simulink model "OML58_Cores"  (R2021b)
settings: Solver=ode4  StartTime=0.0  StopTime=inf  FixedStep=Ts  RelTol=1e-3  EnableMultiTasking=on
PostLoadFcn:
  | Ts = 50e-6;
InitFcn:
  | Ts = 50e-6;
undefined symbols (not defined in the file): I, Left, Right, type, V
libraries: spsSeriesRLCBranchLib x24, spsThreePhaseSeriesRLCLoadLib x12, spsThreePhaseSeriesRLCBranchLib x12, spsThreePhaseBreakerLib x12, artemis x10, spsGroundLib x8, rtlab x6, LafaeLib x6, spsThreePhaseTransformerTwoWindingsLib x5, spsThreePhaseVIMeasurementLib x5, spsPower3phInstantaneousLib x3, spsThreePhaseSourceLib x1
(part 2 of 3)

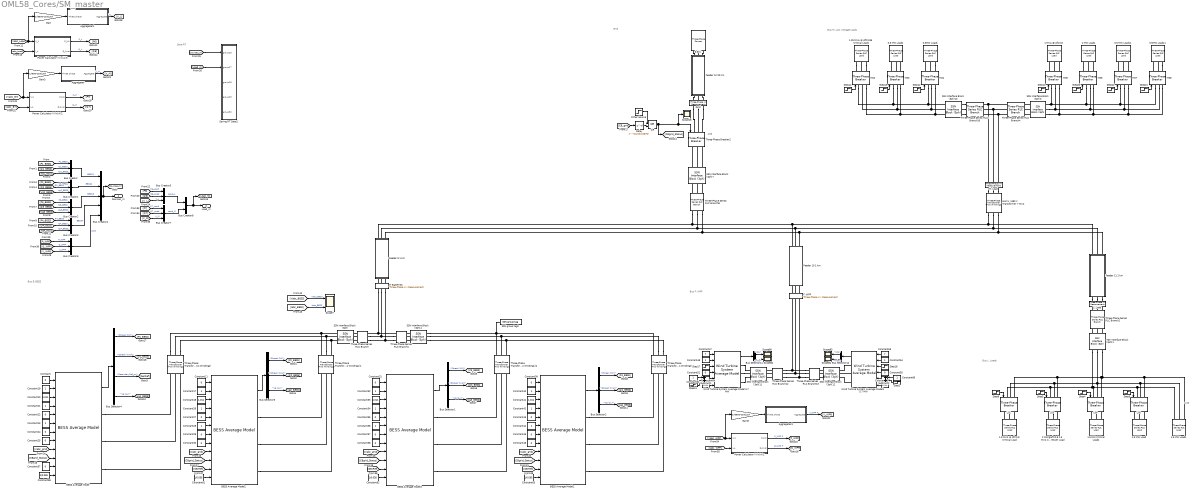
== system OML58_Cores/SM_master ==
  note: Bus E: BESS
  note: L06
  note: Bus L: Loads
  note: Save RT
  note: Grid
  note: A06
  note: Bus M: Low Voltage Loads
  note: Bus F: WPP
  0.5 MW Loads : spsThreePhaseSeriesRLCLoadLib/Three-Phase Series RLC Load  LConnTagsString=A|B|C  Configuration=Y (grounded)  NominalVoltage=690  Vabc=[1e3 1e3 1e3]  Vabcp=[1e3 1e3 1e3]  NominalFrequency=50  UnbalancedPower=off  ActivePower=0.5e06  InductivePower=0  CapacitivePower=0  Pabc=[10e3 9e3 11e3]  QLabc=[100 90 110]  QCabc=[100 90 110]  Pabcp=[10e3 9e3 11e3]  QLabcp=[100 90 110]  QCabcp=[100 90 110]  Measurements=None  LoadType=constant Z
  0.5 MW Loads1 : spsThreePhaseSeriesRLCLoadLib/Three-Phase Series RLC Load  LConnTagsString=A|B|C  Configuration=Y (grounded)  NominalVoltage=690  Vabc=[1e3 1e3 1e3]  Vabcp=[1e3 1e3 1e3]  NominalFrequency=50  UnbalancedPower=off  ActivePower=0.5e06  InductivePower=0  CapacitivePower=0  Pabc=[10e3 9e3 11e3]  QLabc=[100 90 110]  QCabc=[100 90 110]  Pabcp=[10e3 9e3 11e3]  QLabcp=[100 90 110]  QCabcp=[100 90 110]  Measurements=None  LoadType=constant Z
  0.5MW Loads : spsThreePhaseSeriesRLCLoadLib/Three-Phase Series RLC Load  LConnTagsString=A|B|C  Configuration=Y (grounded)  NominalVoltage=690  Vabc=[1e3 1e3 1e3]  Vabcp=[1e3 1e3 1e3]  NominalFrequency=50  UnbalancedPower=off  ActivePower=0.5e06  InductivePower=0  CapacitivePower=0  Pabc=[10e3 9e3 11e3]  QLabc=[100 90 110]  QCabc=[100 90 110]  Pabcp=[10e3 9e3 11e3]  QLabcp=[100 90 110]  QCabcp=[100 90 110]  Measurements=None  LoadType=constant Z
  0.5MW Loads1 : spsThreePhaseSeriesRLCLoadLib/Three-Phase Series RLC Load  LConnTagsString=A|B|C  Configuration=Y (grounded)  NominalVoltage=690  Vabc=[1e3 1e3 1e3]  Vabcp=[1e3 1e3 1e3]  NominalFrequency=50  UnbalancedPower=off  ActivePower=0.5e06  InductivePower=0  CapacitivePower=0  Pabc=[10e3 9e3 11e3]  QLabc=[100 90 110]  QCabc=[100 90 110]  Pabcp=[10e3 9e3 11e3]  QLabcp=[100 90 110]  QCabcp=[100 90 110]  Measurements=None  LoadType=constant Z
  1 MVA @ pf=0.8 : spsThreePhaseSeriesRLCLoadLib/Three-Phase Series RLC Load  LConnTagsString=A|B|C  Configuration=Y (grounded)  NominalVoltage=690  Vabc=[1e3 1e3 1e3]  Vabcp=[1e3 1e3 1e3]  NominalFrequency=50  UnbalancedPower=off  ActivePower=0.8e06  InductivePower=0.6e06  CapacitivePower=0  Pabc=[10e3 9e3 11e3]  QLabc=[100 90 110]  QCabc=[100 90 110]  Pabcp=[10e3 9e3 11e3]  QLabcp=[100 90 110]  QCabcp=[100 90 110]  Measurements=None  LoadType=constant Z
  1 MW Loads : spsThreePhaseSeriesRLCLoadLib/Three-Phase Series RLC Load  LConnTagsString=A|B|C  Configuration=Y (grounded)  NominalVoltage=690  Vabc=[1e3 1e3 1e3]  Vabcp=[1e3 1e3 1e3]  NominalFrequency=50  UnbalancedPower=off  ActivePower=0.5e06  InductivePower=0  CapacitivePower=0  Pabc=[10e3 9e3 11e3]  QLabc=[100 90 110]  QCabc=[100 90 110]  Pabcp=[10e3 9e3 11e3]  QLabcp=[100 90 110]  QCabcp=[100 90 110]  Measurements=None  LoadType=constant Z
  1.25 MVA @ pf=0.85 Critical Loads : spsThreePhaseSeriesRLCLoadLib/Three-Phase Series RLC Load  LConnTagsString=A|B|C  Configuration=Y (grounded)  NominalVoltage=690  Vabc=[1e3 1e3 1e3]  Vabcp=[1e3 1e3 1e3]  NominalFrequency=50  UnbalancedPower=off  ActivePower=1.0625e06  InductivePower=658478  CapacitivePower=0  Pabc=[10e3 9e3 11e3]  QLabc=[100 90 110]  QCabc=[100 90 110]  Pabcp=[10e3 9e3 11e3]  QLabcp=[100 90 110]  QCabcp=[100 90 110]  Measurements=None  LoadType=constant Z
  1.5 MW Critical Loads : spsThreePhaseSeriesRLCLoadLib/Three-Phase Series RLC Load  LConnTagsString=A|B|C  Configuration=Y (grounded)  NominalVoltage=6600  Vabc=[1e3 1e3 1e3]  Vabcp=[1e3 1e3 1e3]  NominalFrequency=50  UnbalancedPower=off  ActivePower=1.5e06  InductivePower=0  CapacitivePower=0  Pabc=[10e3 9e3 11e3]  QLabc=[100 90 110]  QCabc=[100 90 110]  Pabcp=[10e3 9e3 11e3]  QLabcp=[100 90 110]  QCabcp=[100 90 110]  Measurements=None  LoadType=constant Z
  1.5 MW Load : spsThreePhaseSeriesRLCLoadLib/Three-Phase Series RLC Load  LConnTagsString=A|B|C  Configuration=Y (grounded)  NominalVoltage=6600  Vabc=[1e3 1e3 1e3]  Vabcp=[1e3 1e3 1e3]  NominalFrequency=50  UnbalancedPower=off  ActivePower=1.5e06  InductivePower=0  CapacitivePower=0  Pabc=[10e3 9e3 11e3]  QLabc=[100 90 110]  QCabc=[100 90 110]  Pabcp=[10e3 9e3 11e3]  QLabcp=[100 90 110]  QCabcp=[100 90 110]  Measurements=None  LoadType=constant Z
  1.5 MW Loads : spsThreePhaseSeriesRLCLoadLib/Three-Phase Series RLC Load  LConnTagsString=A|B|C  Configuration=Y (grounded)  NominalVoltage=6600  Vabc=[1e3 1e3 1e3]  Vabcp=[1e3 1e3 1e3]  NominalFrequency=50  UnbalancedPower=off  ActivePower=1.5e06  InductivePower=0  CapacitivePower=0  Pabc=[10e3 9e3 11e3]  QLabc=[100 90 110]  QCabc=[100 90 110]  Pabcp=[10e3 9e3 11e3]  QLabcp=[100 90 110]  QCabcp=[100 90 110]  Measurements=None  LoadType=constant Z
  1.9 MVA @ pf=0.9 Critical Load : spsThreePhaseSeriesRLCLoadLib/Three-Phase Series RLC Load  LConnTagsString=A|B|C  Configuration=Y (grounded)  NominalVoltage=6600  Vabc=[1e3 1e3 1e3]  Vabcp=[1e3 1e3 1e3]  NominalFrequency=50  UnbalancedPower=off  ActivePower=1.71e06  InductivePower=828191  CapacitivePower=0  Pabc=[10e3 9e3 11e3]  QLabc=[100 90 110]  QCabc=[100 90 110]  Pabcp=[10e3 9e3 11e3]  QLabcp=[100 90 110]  QCabcp=[100 90 110]  Measurements=None  LoadType=constant Z
  2 MW@pf=0.8 2.5 MVA Compresser Load : spsThreePhaseSeriesRLCLoadLib/Three-Phase Series RLC Load  LConnTagsString=A|B|C  Configuration=Y (grounded)  NominalVoltage=6600  Vabc=[1e3 1e3 1e3]  Vabcp=[1e3 1e3 1e3]  NominalFrequency=50  UnbalancedPower=off  ActivePower=2e06  InductivePower=1.5e06  CapacitivePower=0  Pabc=[10e3 9e3 11e3]  QLabc=[100 90 110]  QCabc=[100 90 110]  Pabcp=[10e3 9e3 11e3]  QLabcp=[100 90 110]  QCabcp=[100 90 110]  Measurements=None  LoadType=constant Z
  "6.6 kV / 690 V Transformer 7 MVA   " : spsThreePhaseTransformerTwoWindingsLib/Three-Phase Transformer (Two Windings)  Winding1Connection=Yg  Winding2Connection=Yg  CoreType=Three single-phase transformers  SetSaturation=off  Hysteresis=off  DataFile='hysteresis'  SetInitialFlux=off  Measurements=None  UNITS=pu  NominalPower=[ 7e6 , 50 ]  Winding1=[ 6.6e3 , 0.03/25 , 0.03 ]  Winding2=[ 690 , 0.03/25 , 0.03 ]  Rm=500  Lm=500  L0=0.5  Saturation=[ 0,0 ; 0.0024,1.2 ; 1.0,1.52 ]  InitialFluxes=[ 0.8 , -0.8 , 0.7 ]  BreakLoop=off  DiscreteSolver=Trapezoidal iterative  DataType=off  TransfoNumber=1
  6.6kV : spsThreePhaseSourceLib/Three-Phase Source  InternalConnection=Yg  VoltagePhases=off  Voltage=6.6e3  PhaseAngle=0  Voltage_phases=[25e3 25e3 25e3]/sqrt(3)  PhaseAngles_phases=[0 -120 +120]  Frequency=50  NonIdealSource=on  SpecifyImpedance=on  Resistance=0.8929  Inductance=16.58e-3  ShortCircuitLevel=50e6*10  BaseVoltage=6.6e3  XRratio=7  BusType=swing  Pref=0  Qref=0  Prefabc=[10e3, 10e3, 10e3]  Qrefabc=[0, 0, 0]  Qmin=-inf  Qmax=inf
  Aggregater : Subsystem
      mask Display: image('$imagefile'); % Use "Edit Image" on toolstrip to change.
  Aggregater1 : Subsystem
      mask Display: image('$imagefile'); % Use "Edit Image" on toolstrip to change.
  Aggregater3 : Subsystem
      mask Display: image('$imagefile'); % Use "Edit Image" on toolstrip to change.
  BESS Average Model : LafaeLib/BESS/BESS Average Model  Vac=690  Vdc=1500  Snom=2.2e6  fnom=50  Capacity=1533  f_switch=6300  fres=720  Ripple=0.05  Kq=0.5  Kv=0.5/0.035  H=0.1  EnbSec=Yes  Ts=Ts
      settings: SourceProductName=LAFAE Library
  BESS Average Model1 : LafaeLib/BESS/BESS Average Model  Vac=690  Vdc=1500  Snom=2.2e6  fnom=50  Capacity=1533  f_switch=6300  fres=720  Ripple=0.05  Kq=0.5  Kv=0.5/0.035  H=0.1  EnbSec=No  Ts=Ts
      settings: SourceProductName=LAFAE Library
  BESS Average Model2 : LafaeLib/BESS/BESS Average Model  Vac=690  Vdc=1500  Snom=2.2e6  fnom=50  Capacity=1533  f_switch=6300  fres=720  Ripple=0.05  Kq=0.5  Kv=0.5/0.035  H=0.1  EnbSec=No  Ts=Ts
      settings: SourceProductName=LAFAE Library
  BESS Average Model3 : LafaeLib/BESS/BESS Average Model  Vac=690  Vdc=1500  Snom=2.2e6  fnom=50  Capacity=1533  f_switch=6300  fres=720  Ripple=0.05  Kq=0.5  Kv=0.5/0.035  H=0.1  EnbSec=No  Ts=Ts
      settings: SourceProductName=LAFAE Library
  Bus Creator{,1..3,5..7} (7 alike) : BusCreator  Inputs=3
  Bus Creator4 : BusCreator  Inputs=5
  Bus Creator8 : BusCreator  Inputs=2
  Bus Selector1 : BusSelector  OutputSignals=Pbreak (kW),Qbreak (kvar),Vg (pu)
  Bus Selector11 : BusSelector  OutputSignals=meas_control.Idq,meas_control.Vdq
  Bus Selector12 : BusSelector  OutputSignals=meas_control.Idq,meas_control.Vdq
  Bus Selector2 : BusSelector  OutputSignals=Pbreak (kW),Qbreak (kvar),Vg (pu)
  Bus Selector4 : BusSelector  OutputSignals=Pbreak (kW),Qbreak (kvar),SecondaryRef_pu,Vg (pu)
  Bus Selector5 : BusSelector  OutputSignals=Pbreak (kW),Qbreak (kvar),Vg (pu)
  Constant{,11,22,24..25,27,29..31,35,37..39,43,45..46,51,55,57} (19 alike) : Constant  Value=0
  Constant{17,19,21,23,26,28,32,34,36,40,42,44,48,52,54,66} (16 alike) : Constant
  Constant{18,20,33,41,64..65} (6 alike) : Constant  Value=1.011
  Constant47 : Constant  Value=7
  Constant53 : Constant  Value=7
  Constant{58,61..63} (4 alike) : Constant  Value=1/0.035
  Delay : Delay  DelayLength=round(0.05/Ts)  SampleTime=Ts
  E: Batteries : spsThreePhaseVIMeasurementLib/Three-Phase V-I Measurement  VoltageMeasurement=phase-to-ground  SetLabelV=on  LabelV=Vabc_BESS  Vpu=off  VpuLL=off  CurrentMeasurement=yes  SetLabelI=on  LabelI=Iabc_BESS  Ipu=off  Pbase=100e6  Vbase=500e3  OutputType=Magnitude  PhasorSimulation=off  PSBequivalent=0
  F: WPP : spsThreePhaseVIMeasurementLib/Three-Phase V-I Measurement  VoltageMeasurement=phase-to-ground  SetLabelV=on  LabelV=Vabc_WPP  Vpu=off  VpuLL=off  CurrentMeasurement=yes  SetLabelI=on  LabelI=Iabc_WPP  Ipu=off  Pbase=100e6  Vbase=500e3  OutputType=Magnitude  PhasorSimulation=off  PSBequivalent=0
  Feeder 10 1 km : Subsystem  mask{l=1}
      mask prompts: l "Comprimento da linha (km)"
      mask DialogControl DescTextVar Prompt: Modelo pi para sequência positiva.
      mask Display: image('$imagefile'); % Use "Edit Image" on toolstrip to change.
  Feeder 11 1 km : Subsystem  mask{l=1}
      mask prompts: l "Comprimento da linha (km)"
      mask DialogControl DescTextVar Prompt: Modelo pi para sequência positiva.
      mask Display: image('$imagefile'); % Use "Edit Image" on toolstrip to change.
  Feeder 12 20 km : Subsystem  mask{l=20}
      mask prompts: l "Comprimento da linha (km)"
      mask DialogControl DescTextVar Prompt: Modelo pi para sequência positiva.
      mask Display: image('$imagefile'); % Use "Edit Image" on toolstrip to change.
  Feeder 9 1 km : Subsystem  mask{l=1}
      mask prompts: l "Comprimento da linha (km)"
      mask DialogControl DescTextVar Prompt: Modelo pi para sequência positiva.
      mask Display: image('$imagefile'); % Use "Edit Image" on toolstrip to change.
  Gain : Gain  Gain=1/(6600*sqrt(2/3))
  Gain3 : Gain  Gain=1/(690*sqrt(2/3))
  Gain8 : Gain  Gain=1/(6600*sqrt(2/3))
  Grid : spsThreePhaseVIMeasurementLib/Three-Phase V-I Measurement  VoltageMeasurement=phase-to-ground  SetLabelV=on  LabelV=Vabc_grid  Vpu=off  VpuLL=off  CurrentMeasurement=yes  SetLabelI=on  LabelI=Iabc_grid  Ipu=off  Pbase=100e6  Vbase=500e3  OutputType=Magnitude  PhasorSimulation=off  PSBequivalent=0
  L02 : spsThreePhaseBreakerLib/Three-Phase Breaker  InitialState=open  SwitchA=on  SwitchB=on  SwitchC=on  SwitchTimes="[1/60  5/60]"  External=on  BreakerResistance=0.01  SnubberResistance=1e8  SnubberCapacitance=inf  Measurements=None
  L03 : spsThreePhaseBreakerLib/Three-Phase Breaker  InitialState=open  SwitchA=on  SwitchB=on  SwitchC=on  SwitchTimes="[1/60  5/60]"  External=on  BreakerResistance=0.01  SnubberResistance=1e8  SnubberCapacitance=inf  Measurements=None
  L04 : spsThreePhaseBreakerLib/Three-Phase Breaker  InitialState=open  SwitchA=on  SwitchB=on  SwitchC=on  SwitchTimes="[1/60  5/60]"  External=on  BreakerResistance=0.01  SnubberResistance=1e8  SnubberCapacitance=inf  Measurements=None
  L05 : spsThreePhaseBreakerLib/Three-Phase Breaker  InitialState=open  SwitchA=on  SwitchB=on  SwitchC=on  SwitchTimes="[1/60  5/60]"  External=on  BreakerResistance=0.01  SnubberResistance=1e8  SnubberCapacitance=inf  Measurements=None
  L: Load : spsThreePhaseVIMeasurementLib/Three-Phase V-I Measurement  VoltageMeasurement=phase-to-ground  SetLabelV=on  LabelV=Vabc_Load  Vpu=off  VpuLL=off  CurrentMeasurement=yes  SetLabelI=on  LabelI=Iabc_Load  Ipu=off  Pbase=100e6  Vbase=500e3  OutputType=Magnitude  PhasorSimulation=off  PSBequivalent=0
  M02 : spsThreePhaseBreakerLib/Three-Phase Breaker  InitialState=open  SwitchA=on  SwitchB=on  SwitchC=on  SwitchTimes="[1/60  5/60]"  External=on  BreakerResistance=0.01  SnubberResistance=1e7  SnubberCapacitance=inf  Measurements=None
  M03 : spsThreePhaseBreakerLib/Three-Phase Breaker  InitialState=open  SwitchA=on  SwitchB=on  SwitchC=on  SwitchTimes="[1/60  5/60]"  External=on  BreakerResistance=0.01  SnubberResistance=1e7  SnubberCapacitance=inf  Measurements=None
  M04 : spsThreePhaseBreakerLib/Three-Phase Breaker  InitialState=open  SwitchA=on  SwitchB=on  SwitchC=on  SwitchTimes="[1/60  5/60]"  External=on  BreakerResistance=0.01  SnubberResistance=1e7  SnubberCapacitance=inf  Measurements=None
  M05 : spsThreePhaseBreakerLib/Three-Phase Breaker  InitialState=open  SwitchA=on  SwitchB=on  SwitchC=on  SwitchTimes="[1/60  5/60]"  External=on  BreakerResistance=0.01  SnubberResistance=1e7  SnubberCapacitance=inf  Measurements=None
  M06 : spsThreePhaseBreakerLib/Three-Phase Breaker  InitialState=open  SwitchA=on  SwitchB=on  SwitchC=on  SwitchTimes="[1/60  5/60]"  External=on  BreakerResistance=0.01  SnubberResistance=1e7  SnubberCapacitance=inf  Measurements=None
  M07 : spsThreePhaseBreakerLib/Three-Phase Breaker  InitialState=open  SwitchA=on  SwitchB=on  SwitchC=on  SwitchTimes="[1/60  5/60]"  External=on  BreakerResistance=0.01  SnubberResistance=1e7  SnubberCapacitance=inf  Measurements=None
  M08 : spsThreePhaseBreakerLib/Three-Phase Breaker  InitialState=open  SwitchA=on  SwitchB=on  SwitchC=on  SwitchTimes="[1/60  5/60]"  External=on  BreakerResistance=0.01  SnubberResistance=1e7  SnubberCapacitance=inf  Measurements=None
  M: Load : spsThreePhaseVIMeasurementLib/Three-Phase V-I Measurement  VoltageMeasurement=phase-to-ground  SetLabelV=on  LabelV=Vabc_B7  Vpu=off  VpuLL=off  CurrentMeasurement=yes  SetLabelI=on  LabelI=Iabc_B7  Ipu=off  Pbase=100e6  Vbase=500e3  OutputType=Magnitude  PhasorSimulation=off  PSBequivalent=0
  OR : Logic  Operator=OR  IconShape=distinctive  AllPortsSameDT=off  OutDataTypeStr=boolean
  Other Source : Step  Time=1000  SampleTime=Ts
  Power Calculator (V)x(A)1 : Subsystem
      mask DialogControl DescTextVar Prompt: Compute the three-phase instantaneous active and reactive powers associated with a periodic set of three-phase voltages and currents.
      mask DialogControl Control2 Prompt: Instantaneous reactive power is accurate only for balanced and harmonic-free three-phase voltages and currents.
      mask DialogControl Control3 Prompt: Current flowing into an RL circuit will produce positive active and reactive power.
      mask DialogControl Control4 Prompt: Input currents and voltages in (A) and (V), respectively.
      mask DialogControl Control5 Prompt: Output P and Q in kW and kvar, respectively.
      mask Display: image('$imagefile'); % Use "Edit Image" on toolstrip to change.
  Power Calculator (V)x(A)2 : Subsystem
      mask DialogControl DescTextVar Prompt: Compute the three-phase instantaneous active and reactive powers associated with a periodic set of three-phase voltages and currents.
      mask DialogControl Control2 Prompt: Instantaneous reactive power is accurate only for balanced and harmonic-free three-phase voltages and currents.
      mask DialogControl Control3 Prompt: Current flowing into an RL circuit will produce positive active and reactive power.
      mask DialogControl Control4 Prompt: Input currents and voltages in (A) and (V), respectively.
      mask DialogControl Control5 Prompt: Output P and Q in kW and kvar, respectively.
      mask Display: image('$imagefile'); % Use "Edit Image" on toolstrip to change.
  Power Calculator (V)x(A)3 : Subsystem
      mask DialogControl DescTextVar Prompt: Compute the three-phase instantaneous active and reactive powers associated with a periodic set of three-phase voltages and currents.
      mask DialogControl Control2 Prompt: Instantaneous reactive power is accurate only for balanced and harmonic-free three-phase voltages and currents.
      mask DialogControl Control3 Prompt: Current flowing into an RL circuit will produce positive active and reactive power.
      mask DialogControl Control4 Prompt: Input currents and voltages in (A) and (V), respectively.
      mask DialogControl Control5 Prompt: Output P and Q in kW and kvar, respectively.
      mask Display: image('$imagefile'); % Use "Edit Image" on toolstrip to change.
  SSN Interface Block (3ph) : artemis/SSN/Nodal Interface Blocks/SSN Interface Block (3ph)  nb_phase=3  nb_port=2  p1_type=V-type(Left)  p2_type=I-type(Right)  p3_type=V-type(Left)  p4_type=V-type(Left)  p5_type=V-type(Left)  p6_type=V-type(Left)  p7_type=V-type(Left)  p8_type=V-type(Left)  p9_type=V-type(Left)  p10_type=V-type(Left)  p11_type=V-type(Left)  p12_type=V-type(Left)  p13_type=V-type(Left)  p14_type=V-type(Left)  p15_type=V-type(Left)  p16_type=V-type(Left)  I_port_shunt_resistance=1e6
  SSN Interface Block (3ph)1 : artemis/SSN/Nodal Interface Blocks/SSN Interface Block (3ph)  nb_phase=3  nb_port=2  p1_type=I-type(Left)  p2_type=V-type (Right)  p3_type=V-type(Left)  p4_type=V-type(Left)  p5_type=V-type(Left)  p6_type=V-type(Left)  p7_type=V-type(Left)  p8_type=V-type(Left)  p9_type=V-type(Left)  p10_type=V-type(Left)  p11_type=V-type(Left)  p12_type=V-type(Left)  p13_type=V-type(Left)  p14_type=V-type(Left)  p15_type=V-type(Left)  p16_type=V-type(Left)  I_port_shunt_resistance=1e6
  SSN Interface Block (3ph)10 : artemis/SSN/Nodal Interface Blocks/SSN Interface Block (3ph)  nb_phase=3  nb_port=2  p1_type=V-type (Right)  p2_type=I-type(Left)  p3_type=V-type(Left)  p4_type=V-type(Left)  p5_type=V-type(Left)  p6_type=V-type(Left)  p7_type=V-type(Left)  p8_type=V-type(Left)  p9_type=V-type(Left)  p10_type=V-type(Left)  p11_type=V-type(Left)  p12_type=V-type(Left)  p13_type=V-type(Left)  p14_type=V-type(Left)  p15_type=V-type(Left)  p16_type=V-type(Left)  I_port_shunt_resistance=1e6
  SSN Interface Block (3ph)11 : artemis/SSN/Nodal Interface Blocks/SSN Interface Block (3ph)  nb_phase=3  nb_port=2  p1_type=I-type(Left)  p2_type=V-type (Right)  p3_type=V-type(Left)  p4_type=V-type(Left)  p5_type=V-type(Left)  p6_type=V-type(Left)  p7_type=V-type(Left)  p8_type=V-type(Left)  p9_type=V-type(Left)  p10_type=V-type(Left)  p11_type=V-type(Left)  p12_type=V-type(Left)  p13_type=V-type(Left)  p14_type=V-type(Left)  p15_type=V-type(Left)  p16_type=V-type(Left)  I_port_shunt_resistance=1e4
  SSN Interface Block (3ph)12 : artemis/SSN/Nodal Interface Blocks/SSN Interface Block (3ph)  nb_phase=3  nb_port=2  p1_type=V-type(Left)  p2_type=I-type(Right)  p3_type=V-type(Left)  p4_type=V-type(Left)  p5_type=V-type(Left)  p6_type=V-type(Left)  p7_type=V-type(Left)  p8_type=V-type(Left)  p9_type=V-type(Left)  p10_type=V-type(Left)  p11_type=V-type(Left)  p12_type=V-type(Left)  p13_type=V-type(Left)  p14_type=V-type(Left)  p15_type=V-type(Left)  p16_type=V-type(Left)  I_port_shunt_resistance=1e4
  SSN Interface Block (3ph)3 : artemis/SSN/Nodal Interface Blocks/SSN Interface Block (3ph)  nb_phase=3  nb_port=2  p1_type=V-type(Left)  p2_type=I-type(Right)  p3_type=V-type(Left)  p4_type=V-type(Left)  p5_type=V-type(Left)  p6_type=V-type(Left)  p7_type=V-type(Left)  p8_type=V-type(Left)  p9_type=V-type(Left)  p10_type=V-type(Left)  p11_type=V-type(Left)  p12_type=V-type(Left)  p13_type=V-type(Left)  p14_type=V-type(Left)  p15_type=V-type(Left)  p16_type=V-type(Left)  I_port_shunt_resistance=1e6
  SSN Interface Block (3ph)4 : artemis/SSN/Nodal Interface Blocks/SSN Interface Block (3ph)  nb_phase=3  nb_port=2  p1_type=V-type(Left)  p2_type=I-type(Right)  p3_type=V-type(Left)  p4_type=V-type(Left)  p5_type=V-type(Left)  p6_type=V-type(Left)  p7_type=V-type(Left)  p8_type=V-type(Left)  p9_type=V-type(Left)  p10_type=V-type(Left)  p11_type=V-type(Left)  p12_type=V-type(Left)  p13_type=V-type(Left)  p14_type=V-type(Left)  p15_type=V-type(Left)  p16_type=V-type(Left)  I_port_shunt_resistance=1e6
  SSN Interface Block (3ph)7 : artemis/SSN/Nodal Interface Blocks/SSN Interface Block (3ph)  nb_phase=3  nb_port=2  p1_type=V-type (Right)  p2_type=I-type(Left)  p3_type=V-type(Left)  p4_type=V-type(Left)  p5_type=V-type(Left)  p6_type=V-type(Left)  p7_type=V-type(Left)  p8_type=V-type(Left)  p9_type=V-type(Left)  p10_type=V-type(Left)  p11_type=V-type(Left)  p12_type=V-type(Left)  p13_type=V-type(Left)  p14_type=V-type(Left)  p15_type=V-type(Left)  p16_type=V-type(Left)  I_port_shunt_resistance=1e6
  SSN group tag2 : artemis/SSN/SSN group tag  ssn_group_tag=BESS2
  Saving RT Data2 : Subsystem  mask{Ts=Ts, Decimation26=2, varname26=BESS_m, Filename26=BESS_m.mat, nls26=15, ld26=65, Decimation27=2, varname27=Load_L, Filename27=Load_L.mat, nls27=6, ld27=65, Decimation28=2, varname28=Meas_Q, Filename28=Meas_Q.mat, nls28=7, ld28=65, Decimation29=2, varname29=P_Loads, Filename29=P_Loads.mat, nls29=4, ld29=65, Decimation30=2, varname30=Q_Loads, Filename30=Q_Loads.mat, nls30=4, ld30=65}
      mask prompts: Ts "Ts (s)"; Decimation26 "Decimation factor"; varname26 "Variable name"; Filename26 "FileName"; nls26 "Number of logged signals"; ld26 "Logging duration (s)"; Decimation27 "Decimation factor"; varname27 "Variable name"; Filename27 "FileName"; nls27 "Number of logged signals"; ld27 "Logging duration (s)"; Decimation28 "Decimation factor"; varname28 "Variable name"; Filename28 "FileName"; nls28 "Number of logged signals"; ld28 "Logging duration (s)"; Decimation29 "Decimation factor"; varname29 "Variable name"; Filename29 "FileName"; nls29 "Number of logged signals"; ld29 "Logging duration (s)"; Decimation30 "Decimation factor"; varname30 "Variable name"; Filename30 "FileName"; nls30 "Number of logged signals"; ld30 "Logging duration (s)"
      mask help: This block contains the 5 groups of OpWriteFile (26, 27, 28 29 and 30) blocks that write signals to a binary file (.mat), files that are in the binary data container format that MATLAB uses.
      mask TypeOptions Decimation26: OpWriteFile26/Decimation
      mask TypeOptions varname26: OpWriteFile26/varname
      mask TypeOptions Filename26: OpWriteFile26/Filename
      mask TypeOptions Decimation27: OpWriteFile27/Decimation
      mask TypeOptions varname27: OpWriteFile27/varname
      mask TypeOptions Filename27: OpWriteFile27/Filename
      mask TypeOptions Decimation28: OpWriteFile28/Decimation
      mask TypeOptions varname28: OpWriteFile28/varname
      mask TypeOptions Filename28: OpWriteFile28/Filename
      mask TypeOptions Decimation29: OpWriteFile29/Decimation
      mask TypeOptions varname29: OpWriteFile29/varname
      mask TypeOptions Filename29: OpWriteFile29/Filename
      mask TypeOptions Decimation30: OpWriteFile30/Decimation
      mask TypeOptions varname30: OpWriteFile30/varname
      mask TypeOptions Filename30: OpWriteFile30/Filename
      mask DialogControl DescGroupVar Prompt: Saving RT Data
      mask DialogControl Container4 Prompt: Group 26
      mask DialogControl Container9 Prompt: Group 27
      mask DialogControl Container10 Prompt: Group 28
      mask DialogControl Container11 Prompt: Group 29
      mask DialogControl Container12 Prompt: Group 30
  Scope{16,80,82..84} (5 alike) : Scope
  Scope7 : Scope  NumInputPorts=2
  Step11 : Step  Time=75  SampleTime=0
  Step12 : Step  Time=12  SampleTime=0
  Step13 : Step  Time=10  SampleTime=0
  Step14 : Step  Time=70  SampleTime=0
  Step17 : Step  Time=3  SampleTime=0
  Step18 : Step  Time=7  SampleTime=0
  Step2 : Step  Time=7.5  SampleTime=0
  Step20 : Step  Time=15  SampleTime=0
  Step21 : Step  Time=25  SampleTime=0
  Step22 : Step  Time=20  SampleTime=0
  Step24 : Step  Time=3.5  SampleTime=0
  Step3 : Step  Time=5  SampleTime=0
  Step4 : Step  Time=2  SampleTime=0
  Step5 : Step  Time=65  SampleTime=0
  Step6 : Step  Time=60  SampleTime=0
  Subtract1 : Sum
  Subtract2 : Sum
  Three-Phase Series RLC Branch{,1..2,4,8,10} (6 alike) : spsThreePhaseSeriesRLCBranchLib/Three-Phase Series RLC Branch  LConnTagsString=A|B|C  RConnTagsString=A|B|C  BranchType=R  Resistance=1e-6  Inductance=1e-3  Capacitance=1e-6  Measurements=None
  Three-Phase Series RLC Branch12 : spsThreePhaseSeriesRLCBranchLib/Three-Phase Series RLC Branch  LConnTagsString=A|B|C  RConnTagsString=A|B|C  BranchType=RL  Resistance=10e-6  Inductance=1e-6  Capacitance=1e-6  Measurements=None
  Three-Phase Series RLC Branch13 : spsThreePhaseSeriesRLCBranchLib/Three-Phase Series RLC Branch  LConnTagsString=A|B|C  RConnTagsString=A|B|C  BranchType=RL  Resistance=10e-6  Inductance=1e-6  Capacitance=1e-6  Measurements=None
  Three-Phase Transformer (Two Windings) : spsThreePhaseTransformerTwoWindingsLib/Three-Phase Transformer (Two Windings)  Winding1Connection=Yg  Winding2Connection=Yg  CoreType=Three single-phase transformers  SetSaturation=off  Hysteresis=off  DataFile='hysteresis'  SetInitialFlux=off  Measurements=None  UNITS=pu  NominalPower=[ 3e6 , 50 ]  Winding1=[ 6.6e3 , 0.03/25 , 0.03 ]  Winding2=[ 690 , 0.03/25 , 0.03 ]  Rm=500  Lm=500  L0=0.5  Saturation=[ 0,0 ; 0.0024,1.2 ; 1.0,1.52 ]  InitialFluxes=[ 0.8 , -0.8 , 0.7 ]  BreakLoop=off  DiscreteSolver=Trapezoidal iterative  DataType=off  TransfoNumber=1
  Three-Phase Transformer (Two Windings)1 : spsThreePhaseTransformerTwoWindingsLib/Three-Phase Transformer (Two Windings)  Winding1Connection=Yg  Winding2Connection=Yg  CoreType=Three single-phase transformers  SetSaturation=off  Hysteresis=off  DataFile='hysteresis'  SetInitialFlux=off  Measurements=None  UNITS=pu  NominalPower=[ 3e6 , 50 ]  Winding1=[ 6.6e3 , 0.03/25 , 0.03 ]  Winding2=[ 690 , 0.03/25 , 0.03 ]  Rm=500  Lm=500  L0=0.5  Saturation=[ 0,0 ; 0.0024,1.2 ; 1.0,1.52 ]  InitialFluxes=[ 0.8 , -0.8 , 0.7 ]  BreakLoop=off  DiscreteSolver=Trapezoidal iterative  DataType=off  TransfoNumber=1
  Three-Phase Transformer (Two Windings)2 : spsThreePhaseTransformerTwoWindingsLib/Three-Phase Transformer (Two Windings)  Winding1Connection=Yg  Winding2Connection=Yg  CoreType=Three single-phase transformers  SetSaturation=off  Hysteresis=off  DataFile='hysteresis'  SetInitialFlux=off  Measurements=None  UNITS=pu  NominalPower=[ 3e6 , 50 ]  Winding1=[ 6.6e3 , 0.03/25 , 0.03 ]  Winding2=[ 690 ,0.03/25 , 0.03 ]  Rm=500  Lm=500  L0=0.5  Saturation=[ 0,0 ; 0.0024,1.2 ; 1.0,1.52 ]  InitialFluxes=[ 0.8 , -0.8 , 0.7 ]  BreakLoop=off  DiscreteSolver=Trapezoidal iterative  DataType=off  TransfoNumber=1
  Three-Phase Transformer (Two Windings)3 : spsThreePhaseTransformerTwoWindingsLib/Three-Phase Transformer (Two Windings)  Winding1Connection=Yg  Winding2Connection=Yg  CoreType=Three single-phase transformers  SetSaturation=off  Hysteresis=off  DataFile='hysteresis'  SetInitialFlux=off  Measurements=None  UNITS=pu  NominalPower=[ 3e6 , 50 ]  Winding1=[ 6.6e3 , 0.03/25 , 0.03 ]  Winding2=[ 690 , 0.03/25 , 0.03 ]  Rm=500  Lm=500  L0=0.5  Saturation=[ 0,0 ; 0.0024,1.2 ; 1.0,1.52 ]  InitialFluxes=[ 0.8 , -0.8 , 0.7 ]  BreakLoop=off  DiscreteSolver=Trapezoidal iterative  DataType=off  TransfoNumber=1
  Three-Phase Breaker2 : spsThreePhaseBreakerLib/Three-Phase Breaker  InitialState=open  SwitchA=on  SwitchB=on  SwitchC=on  SwitchTimes="[1/60  5/60]"  External=on  BreakerResistance=0.01  SnubberResistance=1e8  SnubberCapacitance=inf  Measurements=None
  Wind Turbine System Average Model 5.7 MW : LafaeLib/Wind Turbine/Wind Turbine System Average Model  Pnom=5.7e6  FP=0.95  f=50  fsw_inv=126*50  Vnom_high=6.6e3  Vnom_rms=690  m=0.7  a=2  Droop_V=3.5  Droop_f=10  tau_i=5e-3  ripple_inv=0.1  damp=50  fres=720  ripple_Vdc=0.001  R1=0.03/25  L1=0.03  R2=0.03/25  L2=0.03  Rm=500  Lm=500  Ts=Ts
      settings: SourceProductName=LAFAE Library
  Wind Turbine System Average Model1 5.7 MW : LafaeLib/Wind Turbine/Wind Turbine System Average Model  Pnom=5.7e6  FP=0.95  f=50  fsw_inv=126*50  Vnom_high=6.6e3  Vnom_rms=690  m=0.7  a=2  Droop_V=3.5  Droop_f=10  tau_i=1e-3  ripple_inv=0.1  damp=50  fres=720  ripple_Vdc=0.001  R1=0.03/25  L1=0.03  R2=0.03/25  L2=0.03  Rm=500  Lm=500  Ts=Ts
      settings: SourceProductName=LAFAE Library
  Sources_m : Outport
  Load_m : Outport  Port=2
  wires:
  Constant36/1 -> BESS Average Model3/6
  Constant11/1 -> BESS Average Model2/1
  [CBgrid_Status] -> BESS Average Model2/10
  Constant41/1 -> BESS Average Model1/3
  Constant63/1 -> BESS Average Model1/12
  [CBgrid_Status] -> BESS Average Model3/10
  Constant42/1 -> BESS Average Model1/4
  Constant62/1 -> BESS Average Model3/12
  [Vabc_grid] -> BESS Average Model2/9
  Bus Selector4/1 -> [P1_BESS]  "<Pbreak (kW)>"
  Constant40/1 -> BESS Average Model1/2
  Constant27/1 -> BESS Average Model2/5
  Constant35/1 -> BESS Average Model3/5
  BESS Average Model2/1 -> Bus Selector5/1
  [Vabc_grid] -> BESS Average Model1/9
  Constant43/1 -> BESS Average Model1/5
  Constant17/1 -> BESS Average Model2/2
  [Iabc_BESS] -> Scope7/2  "Iabc_BESS"
  [Vabc_BESS] -> Scope7/1  "Vabc_BESS"
  Constant32/1 -> BESS Average Model3/2
  Bus Selector4/2 -> [Q1_BESS]  "<Qbreak (kvar)>"
  Constant30/1 -> BESS Average Model2/8
  Constant45/1 -> BESS Average Model1/7
  Constant33/1 -> BESS Average Model3/3
  [SecRef] -> BESS Average Model1/11
  Constant18/1 -> BESS Average Model2/3
  Constant31/1 -> BESS Average Model3/1
  Constant28/1 -> BESS Average Model2/6
  Constant29/1 -> BESS Average Model2/7
  Constant26/1 -> BESS Average Model2/4
  [Vabc_grid] -> BESS Average Model3/9
  Bus Selector4/4 -> [Vg1_BESS]  "<Vg (pu)>"
  Constant37/1 -> BESS Average Model3/7
  Constant44/1 -> BESS Average Model1/6
  Constant38/1 -> BESS Average Model3/8
  Constant34/1 -> BESS Average Model3/4
  Constant61/1 -> BESS Average Model2/12
  Bus Selector4/3 -> [SecRef]  "<SecondaryRef_pu>"
  Constant46/1 -> BESS Average Model1/8
  [SecRef] -> BESS Average Model2/11
  [SecRef] -> BESS Average Model3/11
  [CBgrid_Status] -> BESS Average Model1/10
  Constant39/1 -> BESS Average Model1/1
  BESS Average Model/1 -> Bus Selector4/1
  Step3/1 -> L05/1
  Step6/1 -> L02/1
  Step5/1 -> L03/1
  Step4/1 -> L04/1
  Bus Selector5/1 -> [P2_BESS]  "<Pbreak (kW)>"
  Bus Selector5/2 -> [Q2_BESS]  "<Qbreak (kvar)>"
  Bus Selector5/3 -> [Vg2_BESS]  "<Vg (pu)>"
  Bus Selector1/3 -> [Vg3_BESS]  "<Vg (pu)>"
  Bus Selector1/2 -> [Q3_BESS]  "<Qbreak (kvar)>"
  Bus Selector1/1 -> [P3_BESS]  "<Pbreak (kW)>"
  BESS Average Model3/1 -> Bus Selector1/1
  Bus Selector2/1 -> [P4_BESS]  "<Pbreak (kW)>"
  Bus Selector2/2 -> [Q4_BESS]  "<Qbreak (kvar)>"
  Bus Selector2/3 -> [Vg4_BESS]  "<Vg (pu)>"
  BESS Average Model1/1 -> Bus Selector2/1
  [Q1_BESS] -> Bus Creator/2  "Q1_BESS"
  [P1_BESS] -> Bus Creator/1  "P1_BESS"
  [Vg1_BESS] -> Bus Creator/3  "Vg1_BESS"
  [Vg2_BESS] -> Bus Creator1/3  "Vg2_BESS"
  [P2_BESS] -> Bus Creator1/1  "P2_BESS"
  [Q2_BESS] -> Bus Creator1/2  "Q2_BESS"
  [Q4_BESS] -> Bus Creator3/2  "Q4_BESS"
  [P4_BESS] -> Bus Creator3/1  "P4_BESS"
  [Vg4_BESS] -> Bus Creator3/3  "Vg4_BESS"
  [Vg3_BESS] -> Bus Creator2/3  "Vg3_BESS"
  [P3_BESS] -> Bus Creator2/1  "P3_BESS"
  [Q3_BESS] -> Bus Creator2/2  "Q3_BESS"
  Bus Creator/1 -> Bus Creator4/1  "BESS1"
  Bus Creator1/1 -> Bus Creator4/2  "BESS2"
  Bus Creator2/1 -> Bus Creator4/3  "BESS3"
  Bus Creator3/1 -> Bus Creator4/4  "BESS4"
  Bus Creator4/1 -> [Sources_m], Sources_m/1
  Power Calculator (V)x(A)3/2(Q_kvar) -> [Q6]  "Q_L"
  Power Calculator (V)x(A)3/1(P_kW) -> [P6]  "P_L"
  [Iabc_Load] -> Power Calculator (V)x(A)3/2(I_A)
  Aggregater1/1(Aggregate) -> [V_L]  "VL"
  Gain/1 -> Aggregater1/1(Three phase)
  [Vabc_Load] -> Power Calculator (V)x(A)3/1(V_V), Gain/1
  [Q6] -> Bus Creator5/2  "Q6_Load"
  [P6] -> Bus Creator5/1  "P6_Load"
  [V_L] -> Bus Creator5/3  "V_L"
  [Sources_m] -> Saving RT Data2/1(group26)
  [Load_m] -> Saving RT Data2/2(group27)
  OR/1 -> Three-Phase Breaker2/1, Scope16/1, [CBgrid_Status]
  [CB_grid] -> Delay/1
  Other Source/1 -> OR/1
  Delay/1 -> OR/2
  Step20/1 -> M06/1
  Step12/1 -> M04/1
  Step22/1 -> M07/1
  Step14/1 -> M02/1
  Step11/1 -> M05/1
  Step21/1 -> M08/1
  Step13/1 -> M03/1
  Constant20/1 -> BESS Average Model/3
  Constant/1 -> BESS Average Model/1
  Constant58/1 -> BESS Average Model/12
  [Vabc_grid] -> BESS Average Model/9
  Constant21/1 -> BESS Average Model/4
  Constant23/1 -> BESS Average Model/6
  Constant25/1 -> BESS Average Model/8
  Constant24/1 -> BESS Average Model/7
  [CBgrid_Status] -> BESS Average Model/10
  Constant19/1 -> BESS Average Model/2
  Constant57/1 -> BESS Average Model/11
  Constant22/1 -> BESS Average Model/5
  Bus Selector12/2 -> Scope84/1  "<Vdq>"
  Power Calculator (V)x(A)1/2(Q_kvar) -> [Q_WPP]  "Q_WPP F"
  Bus Selector11/2 -> Scope82/1  "<Vdq>"
  Constant55/1 -> Wind Turbine System Average Model1 5.7 MW/4
  [Vabc_WPP] -> Power Calculator (V)x(A)1/1(V_V), Gain8/1
  Wind Turbine System Average Model 5.7 MW/1 -> Bus Selector11/1
  Aggregater3/1(Aggregate) -> [V_WPP]  "V_WPP F"
  Constant48/1 -> Wind Turbine System Average Model 5.7 MW/2
  Constant53/1 -> Wind Turbine System Average Model1 5.7 MW/1
  Step17/1 -> Wind Turbine System Average Model 5.7 MW/3
  Constant54/1 -> Wind Turbine System Average Model1 5.7 MW/2
  Step18/1 -> Wind Turbine System Average Model1 5.7 MW/3
  Subtract2/1 -> Wind Turbine System Average Model1 5.7 MW/5
  Constant51/1 -> Wind Turbine System Average Model 5.7 MW/4
  Constant66/1 -> Subtract2/1
  Step2/1 -> Subtract2/2
  Constant52/1 -> Subtract1/1
  Subtract1/1 -> Wind Turbine System Average Model 5.7 MW/5
  Bus Selector12/1 -> Scope83/1  "<Idq>"
  Constant64/1 -> Wind Turbine System Average Model 5.7 MW/6
  Constant47/1 -> Wind Turbine System Average Model 5.7 MW/1
  Wind Turbine System Average Model1 5.7 MW/1 -> Bus Selector12/1
  Constant65/1 -> Wind Turbine System Average Model1 5.7 MW/6
  Bus Selector11/1 -> Scope80/1  "<Idq>"
  [Iabc_WPP] -> Power Calculator (V)x(A)1/2(I_A)
  Power Calculator (V)x(A)1/1(P_kW) -> [P_WPP]  "P_WPP F"
  Step24/1 -> Subtract1/2
  Gain8/1 -> Aggregater3/1(Three phase)
  [P_WPP] -> Bus Creator6/1  "P_WPP"
  [Q_WPP] -> Bus Creator6/2  "Q_WPP"
  [V_WPP] -> Bus Creator6/3  "V_WPP"
  Bus Creator6/1 -> Bus Creator4/5  "WPP"
  Gain3/1 -> Aggregater/1(Three phase)
  Power Calculator (V)x(A)2/1(P_kW) -> [P7]  "P_M"
  [Iabc_B7] -> Power Calculator (V)x(A)2/2(I_A)
  [Vabc_B7] -> Power Calculator (V)x(A)2/1(V_V), Gain3/1
  Power Calculator (V)x(A)2/2(Q_kvar) -> [Q7]  "Q_M"
  Aggregater/1(Aggregate) -> [V_M]  "V_M"
  [P7] -> Bus Creator7/1  "P7_Load"
  [Q7] -> Bus Creator7/2  "Q7_Load"
  [V_M] -> Bus Creator7/3  "V_M"
  Bus Creator5/1 -> Bus Creator8/1  "Load_L"
  Bus Creator7/1 -> Bus Creator8/2  "Load_M"
  Bus Creator8/1 -> [Load_m], Load_m/1
  connections:
  Three-Phase Series RLC Branch1/LConn3 -- Three-Phase Series RLC Branch/LConn3 -- E: Batteries/RConn3
  Three-Phase Series RLC Branch/LConn1 -- E: Batteries/RConn1 -- Three-Phase Series RLC Branch1/LConn1
  Three-Phase Transformer (Two Windings)3/LConn2 -- Three-Phase Transformer (Two Windings)2/LConn2 -- SSN Interface Block (3ph)4/RConn2
  Three-Phase Transformer (Two Windings)/LConn1 -- Three-Phase Transformer (Two Windings)1/LConn1 -- SSN Interface Block (3ph)/RConn1
  Three-Phase Series RLC Branch1/LConn2 -- Three-Phase Series RLC Branch/LConn2 -- E: Batteries/RConn2
  Three-Phase Transformer (Two Windings)1/LConn2 -- Three-Phase Transformer (Two Windings)/LConn2 -- SSN Interface Block (3ph)/RConn2
  Three-Phase Transformer (Two Windings)/LConn3 -- Three-Phase Transformer (Two Windings)1/LConn3 -- SSN Interface Block (3ph)/RConn3
  Three-Phase Transformer (Two Windings)3/LConn3 -- Three-Phase Transformer (Two Windings)2/LConn3 -- SSN Interface Block (3ph)4/RConn3
  Three-Phase Transformer (Two Windings)2/LConn1 -- SSN group tag2/LConn1 -- SSN Interface Block (3ph)4/RConn1 -- Three-Phase Transformer (Two Windings)3/LConn1
  SSN Interface Block (3ph)4/LConn2 -- Three-Phase Series RLC Branch1/RConn2
  BESS Average Model2/RConn3 -- Three-Phase Transformer (Two Windings)1/RConn3
  E: Batteries/LConn1 -- Feeder 9 1 km/LConn1
  Three-Phase Series RLC Branch1/RConn1 -- SSN Interface Block (3ph)4/LConn1
  BESS Average Model2/RConn1 -- Three-Phase Transformer (Two Windings)1/RConn1
  BESS Average Model1/RConn3 -- Three-Phase Transformer (Two Windings)3/RConn3
  BESS Average Model2/RConn2 -- Three-Phase Transformer (Two Windings)1/RConn2
  SSN Interface Block (3ph)/LConn1 -- Three-Phase Series RLC Branch/RConn1
  SSN Interface Block (3ph)/LConn3 -- Three-Phase Series RLC Branch/RConn3
  SSN Interface Block (3ph)4/LConn3 -- Three-Phase Series RLC Branch1/RConn3
  BESS Average Model/RConn2 -- Three-Phase Transformer (Two Windings)/RConn2
  E: Batteries/LConn3 -- Feeder 9 1 km/LConn3
  BESS Average Model3/RConn1 -- Three-Phase Transformer (Two Windings)2/RConn1
  BESS Average Model1/RConn1 -- Three-Phase Transformer (Two Windings)3/RConn1
  BESS Average Model3/RConn2 -- Three-Phase Transformer (Two Windings)2/RConn2
  BESS Average Model/RConn3 -- Three-Phase Transformer (Two Windings)/RConn3
  BESS Average Model3/RConn3 -- Three-Phase Transformer (Two Windings)2/RConn3
  BESS Average Model/RConn1 -- Three-Phase Transformer (Two Windings)/RConn1
  SSN Interface Block (3ph)/LConn2 -- Three-Phase Series RLC Branch/RConn2
  BESS Average Model1/RConn2 -- Three-Phase Transformer (Two Windings)3/RConn2
  E: Batteries/LConn2 -- Feeder 9 1 km/LConn2
  L03/LConn1 -- L02/LConn1 -- L05/LConn1 -- 1.5 MW Loads/LConn1 -- L04/LConn1 -- SSN Interface Block (3ph)1/LConn1
  L05/LConn3 -- SSN Interface Block (3ph)1/LConn3 -- L02/LConn3 -- L03/LConn3 -- L04/LConn3 -- 1.5 MW Loads/LConn3
  L04/LConn2 -- L05/LConn2 -- 1.5 MW Loads/LConn2 -- SSN Interface Block (3ph)1/LConn2 -- L02/LConn2 -- L03/LConn2
  1.9 MVA @ pf=0.9 Critical Load/LConn3 -- L02/RConn3
  2 MW@pf=0.8 2.5 MVA Compresser Load/LConn3 -- L03/RConn3
  SSN Interface Block (3ph)1/RConn2 -- Three-Phase Series RLC Branch2/RConn2
  SSN Interface Block (3ph)1/RConn3 -- Three-Phase Series RLC Branch2/RConn3
  1.5 MW Load/LConn2 -- L05/RConn2
  Feeder 11 1 km/LConn1 -- L: Load/LConn1
  Three-Phase Series RLC Branch2/LConn2 -- L: Load/RConn2
  1.5 MW Critical Loads/LConn3 -- L04/RConn3
  2 MW@pf=0.8 2.5 MVA Compresser Load/LConn1 -- L03/RConn1
  1.5 MW Critical Loads/LConn1 -- L04/RConn1
  1.9 MVA @ pf=0.9 Critical Load/LConn1 -- L02/RConn1
  1.9 MVA @ pf=0.9 Critical Load/LConn2 -- L02/RConn2
  L03/RConn2 -- 2 MW@pf=0.8 2.5 MVA Compresser Load/LConn2
  Feeder 11 1 km/LConn2 -- L: Load/LConn2
  Three-Phase Series RLC Branch2/LConn1 -- L: Load/RConn1
  SSN Interface Block (3ph)1/RConn1 -- Three-Phase Series RLC Branch2/RConn1
  1.5 MW Load/LConn3 -- L05/RConn3
  Three-Phase Series RLC Branch2/LConn3 -- L: Load/RConn3
  Feeder 11 1 km/LConn3 -- L: Load/LConn3
  1.5 MW Critical Loads/LConn2 -- L04/RConn2
  1.5 MW Load/LConn1 -- L05/RConn1
  Feeder 9 1 km/RConn1 -- Three-Phase Series RLC Branch8/LConn1 -- Feeder 10 1 km/RConn1 -- "6.6 kV / 690 V Transformer 7 MVA   "/LConn1 -- Feeder 11 1 km/RConn1
  Feeder 9 1 km/RConn2 -- Three-Phase Series RLC Branch8/LConn2 -- Feeder 10 1 km/RConn2 -- "6.6 kV / 690 V Transformer 7 MVA   "/LConn2 -- Feeder 11 1 km/RConn2
  Feeder 9 1 km/RConn3 -- Three-Phase Series RLC Branch8/LConn3 -- Feeder 10 1 km/RConn3 -- "6.6 kV / 690 V Transformer 7 MVA   "/LConn3 -- Feeder 11 1 km/RConn3
  6.6kV/RConn2 -- Feeder 12 20 km/RConn2
  Grid/LConn3 -- Three-Phase Breaker2/LConn3
  6.6kV/RConn3 -- Feeder 12 20 km/RConn3
  Three-Phase Series RLC Branch8/RConn1 -- SSN Interface Block (3ph)7/RConn1
  Grid/RConn2 -- Feeder 12 20 km/LConn2
  Three-Phase Series RLC Branch8/RConn2 -- SSN Interface Block (3ph)7/RConn2
  Grid/LConn1 -- Three-Phase Breaker2/LConn1
  Grid/RConn3 -- Feeder 12 20 km/LConn3
  SSN Interface Block (3ph)7/LConn3 -- Three-Phase Breaker2/RConn3
  SSN Interface Block (3ph)7/LConn2 -- Three-Phase Breaker2/RConn2
  Grid/RConn1 -- Feeder 12 20 km/LConn1
  Three-Phase Series RLC Branch8/RConn3 -- SSN Interface Block (3ph)7/RConn3
  SSN Interface Block (3ph)7/LConn1 -- Three-Phase Breaker2/RConn1
  Grid/LConn2 -- Three-Phase Breaker2/LConn2
  6.6kV/RConn1 -- Feeder 12 20 km/RConn1
  SSN Interface Block (3ph)3/RConn2 -- M08/LConn2 -- M07/LConn2 -- M06/LConn2 -- M05/LConn2
  M03/LConn1 -- SSN Interface Block (3ph)10/LConn1 -- M04/LConn1 -- M02/LConn1
  SSN Interface Block (3ph)10/LConn2 -- M04/LConn2 -- M02/LConn2 -- M03/LConn2
  M: Load/RConn3 -- Three-Phase Series RLC Branch10/LConn3 -- Three-Phase Series RLC Branch4/LConn3
  SSN Interface Block (3ph)10/LConn3 -- M04/LConn3 -- M02/LConn3 -- M03/LConn3
  M08/LConn1 -- M07/LConn1 -- M05/LConn1 -- SSN Interface Block (3ph)3/RConn1 -- M06/LConn1
  M: Load/RConn2 -- Three-Phase Series RLC Branch10/LConn2 -- Three-Phase Series RLC Branch4/LConn2
  M: Load/RConn1 -- Three-Phase Series RLC Branch10/LConn1 -- Three-Phase Series RLC Branch4/LConn1
  M06/LConn3 -- M05/LConn3 -- SSN Interface Block (3ph)3/RConn3 -- M08/LConn3 -- M07/LConn3
  M05/RConn2 -- 1 MVA @ pf=0.8/LConn2
  M05/RConn1 -- 1 MVA @ pf=0.8/LConn1
  M07/RConn3 -- 0.5 MW Loads1/LConn3
  M: Load/LConn3 -- "6.6 kV / 690 V Transformer 7 MVA   "/RConn3
  M: Load/LConn2 -- "6.6 kV / 690 V Transformer 7 MVA   "/RConn2
  1.25 MVA @ pf=0.85 Critical Loads/LConn3 -- M02/RConn3
  M07/RConn2 -- 0.5 MW Loads1/LConn2
  M08/RConn2 -- 0.5MW Loads1/LConn2
  M03/RConn2 -- 0.5 MW Loads/LConn2
  M04/RConn1 -- 0.5MW Loads/LConn1
  M02/RConn2 -- 1.25 MVA @ pf=0.85 Critical Loads/LConn2
  1.25 MVA @ pf=0.85 Critical Loads/LConn1 -- M02/RConn1
  M06/RConn3 -- 1 MW Loads/LConn3
  M07/RConn1 -- 0.5 MW Loads1/LConn1
  M03/RConn3 -- 0.5 MW Loads/LConn3
  SSN Interface Block (3ph)3/LConn2 -- Three-Phase Series RLC Branch4/RConn2
  0.5MW Loads/LConn3 -- M04/RConn3
  M03/RConn1 -- 0.5 MW Loads/LConn1
  SSN Interface Block (3ph)10/RConn2 -- Three-Phase Series RLC Branch10/RConn2
  M05/RConn3 -- 1 MVA @ pf=0.8/LConn3
  SSN Interface Block (3ph)3/LConn1 -- Three-Phase Series RLC Branch4/RConn1
  M06/RConn2 -- 1 MW Loads/LConn2
  M06/RConn1 -- 1 MW Loads/LConn1
  SSN Interface Block (3ph)10/RConn3 -- Three-Phase Series RLC Branch10/RConn3
  SSN Interface Block (3ph)10/RConn1 -- Three-Phase Series RLC Branch10/RConn1
  0.5MW Loads1/LConn3 -- M08/RConn3
  M: Load/LConn1 -- "6.6 kV / 690 V Transformer 7 MVA   "/RConn1
  M04/RConn2 -- 0.5MW Loads/LConn2
  SSN Interface Block (3ph)3/LConn3 -- Three-Phase Series RLC Branch4/RConn3
  M08/RConn1 -- 0.5MW Loads1/LConn1
  Three-Phase Series RLC Branch13/LConn2 -- Three-Phase Series RLC Branch12/LConn2 -- F: WPP/LConn2
  Three-Phase Series RLC Branch13/LConn1 -- Three-Phase Series RLC Branch12/LConn1 -- F: WPP/LConn1
  Three-Phase Series RLC Branch13/LConn3 -- Three-Phase Series RLC Branch12/LConn3 -- F: WPP/LConn3
  Three-Phase Series RLC Branch12/RConn2 -- SSN Interface Block (3ph)11/RConn2
  F: WPP/RConn3 -- Feeder 10 1 km/LConn3
  Three-Phase Series RLC Branch12/RConn3 -- SSN Interface Block (3ph)11/RConn3
  F: WPP/RConn1 -- Feeder 10 1 km/LConn1
  F: WPP/RConn2 -- Feeder 10 1 km/LConn2
  Wind Turbine System Average Model1 5.7 MW/RConn3 -- SSN Interface Block (3ph)12/RConn3
  SSN Interface Block (3ph)12/LConn2 -- Three-Phase Series RLC Branch13/RConn2
  Wind Turbine System Average Model1 5.7 MW/RConn1 -- SSN Interface Block (3ph)12/RConn1
  Wind Turbine System Average Model1 5.7 MW/RConn2 -- SSN Interface Block (3ph)12/RConn2
  SSN Interface Block (3ph)12/LConn1 -- Three-Phase Series RLC Branch13/RConn1
  Wind Turbine System Average Model 5.7 MW/RConn1 -- SSN Interface Block (3ph)11/LConn1
  Wind Turbine System Average Model 5.7 MW/RConn2 -- SSN Interface Block (3ph)11/LConn2
  Three-Phase Series RLC Branch12/RConn1 -- SSN Interface Block (3ph)11/RConn1
  SSN Interface Block (3ph)12/LConn3 -- Three-Phase Series RLC Branch13/RConn3
  Wind Turbine System Average Model 5.7 MW/RConn3 -- SSN Interface Block (3ph)11/LConn3

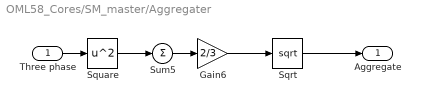
== system OML58_Cores/SM_master/Aggregater ==
  Three phase : Inport
  Gain6 : Gain  Gain=2/3
  Sqrt : Sqrt  SaturateOnIntegerOverflow=on
  Square : Math  Operator=square  SaturateOnIntegerOverflow=on
  Sum5 : Sum  Inputs=1  CollapseMode=Specified dimension
  Aggregate : Outport
  wires:
  Gain6/1 -> Sqrt/1
  Sum5/1 -> Gain6/1
  Square/1 -> Sum5/1
  Sqrt/1 -> Aggregate/1
  Three phase/1 -> Square/1

== system OML58_Cores/SM_master/Aggregater1 ==
  Three phase : Inport
  Gain6 : Gain  Gain=2/3
  Sqrt : Sqrt  SaturateOnIntegerOverflow=on
  Square : Math  Operator=square  SaturateOnIntegerOverflow=on
  Sum5 : Sum  Inputs=1  CollapseMode=Specified dimension
  Aggregate : Outport
  wires:
  Gain6/1 -> Sqrt/1
  Sum5/1 -> Gain6/1
  Square/1 -> Sum5/1
  Sqrt/1 -> Aggregate/1
  Three phase/1 -> Square/1

== system OML58_Cores/SM_master/Aggregater3 ==
  Three phase : Inport
  Gain6 : Gain  Gain=2/3
  Sqrt : Sqrt  SaturateOnIntegerOverflow=on
  Square : Math  Operator=square  SaturateOnIntegerOverflow=on
  Sum5 : Sum  Inputs=1  CollapseMode=Specified dimension
  Aggregate : Outport
  wires:
  Gain6/1 -> Sqrt/1
  Sum5/1 -> Gain6/1
  Square/1 -> Sum5/1
  Sqrt/1 -> Aggregate/1
  Three phase/1 -> Square/1

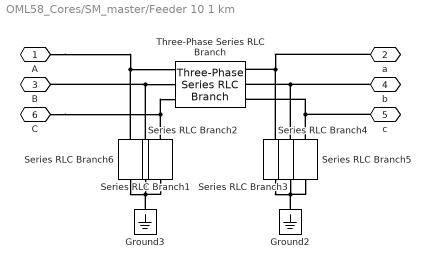
== system OML58_Cores/SM_master/Feeder 10 1 km ==
  Ground2 : spsGroundLib/Ground  LConnTagsString=a
  Ground3 : spsGroundLib/Ground  LConnTagsString=a
  Series RLC Branch{1..6} (6 alike) : spsSeriesRLCBranchLib/Series RLC Branch  LConnTagsString=__new0  RConnTagsString=__new0  BranchType=C  Resistance=1  Inductance=1e-3  SetiL0=off  InitialCurrent=0  Capacitance=l*0.495e-6/2  Setx0=off  InitialVoltage=0  Measurements=None
  Three-Phase Series RLC Branch : spsThreePhaseSeriesRLCBranchLib/Three-Phase Series RLC Branch  LConnTagsString=A|B|C  RConnTagsString=A|B|C  BranchType=RL  Resistance=l*0.0991  Inductance=l*0.602e-3  Capacitance=1e-6  Measurements=None
  A : PMIOPort  Side=Left
  a : PMIOPort  Port=2  Side=Right
  B : PMIOPort  Port=3  Side=Left
  b : PMIOPort  Port=4  Side=Right
  c : PMIOPort  Port=5  Side=Right
  C : PMIOPort  Port=6  Side=Left
  connections:
  Ground2/LConn1 -- Series RLC Branch5/RConn1 -- Series RLC Branch4/RConn1 -- Series RLC Branch3/RConn1
  Series RLC Branch2/LConn1 -- C/RConn1 -- Three-Phase Series RLC Branch/LConn3
  Ground3/LConn1 -- Series RLC Branch2/RConn1 -- Series RLC Branch1/RConn1 -- Series RLC Branch6/RConn1
  Series RLC Branch3/LConn1 -- a/RConn1 -- Three-Phase Series RLC Branch/RConn1
  Series RLC Branch6/LConn1 -- A/RConn1 -- Three-Phase Series RLC Branch/LConn1
  Series RLC Branch4/LConn1 -- b/RConn1 -- Three-Phase Series RLC Branch/RConn2
  Series RLC Branch5/LConn1 -- c/RConn1 -- Three-Phase Series RLC Branch/RConn3
  Series RLC Branch1/LConn1 -- B/RConn1 -- Three-Phase Series RLC Branch/LConn2

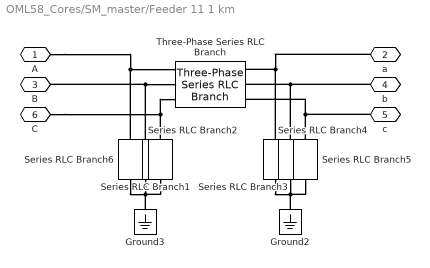
== system OML58_Cores/SM_master/Feeder 11 1 km ==
  Ground2 : spsGroundLib/Ground  LConnTagsString=a
  Ground3 : spsGroundLib/Ground  LConnTagsString=a
  Series RLC Branch{1..6} (6 alike) : spsSeriesRLCBranchLib/Series RLC Branch  LConnTagsString=__new0  RConnTagsString=__new0  BranchType=C  Resistance=1  Inductance=1e-3  SetiL0=off  InitialCurrent=0  Capacitance=l*0.495e-6/2  Setx0=off  InitialVoltage=0  Measurements=None
  Three-Phase Series RLC Branch : spsThreePhaseSeriesRLCBranchLib/Three-Phase Series RLC Branch  LConnTagsString=A|B|C  RConnTagsString=A|B|C  BranchType=RL  Resistance=l*0.0991  Inductance=l*0.602e-3  Capacitance=1e-6  Measurements=None
  A : PMIOPort  Side=Left
  a : PMIOPort  Port=2  Side=Right
  B : PMIOPort  Port=3  Side=Left
  b : PMIOPort  Port=4  Side=Right
  c : PMIOPort  Port=5  Side=Right
  C : PMIOPort  Port=6  Side=Left
  connections:
  Ground2/LConn1 -- Series RLC Branch5/RConn1 -- Series RLC Branch4/RConn1 -- Series RLC Branch3/RConn1
  Series RLC Branch2/LConn1 -- C/RConn1 -- Three-Phase Series RLC Branch/LConn3
  Ground3/LConn1 -- Series RLC Branch2/RConn1 -- Series RLC Branch1/RConn1 -- Series RLC Branch6/RConn1
  Series RLC Branch3/LConn1 -- a/RConn1 -- Three-Phase Series RLC Branch/RConn1
  Series RLC Branch6/LConn1 -- A/RConn1 -- Three-Phase Series RLC Branch/LConn1
  Series RLC Branch4/LConn1 -- b/RConn1 -- Three-Phase Series RLC Branch/RConn2
  Series RLC Branch5/LConn1 -- c/RConn1 -- Three-Phase Series RLC Branch/RConn3
  Series RLC Branch1/LConn1 -- B/RConn1 -- Three-Phase Series RLC Branch/LConn2
